simulink model "TractionControl"  (R2024b)
settings: Solver=FixedStepAuto  StartTime=0.0  StopTime=10.0  RelTol=1e-3  EnableMultiTasking=on
undefined symbols (not defined in the file): Ki1, rStraightSlipRatio, tSlipRatioDerivativeFilterCutoff, tTorqueControlTask
libraries: simulink x9
settings Model: DataDictionary=Master_Dictionary.sldd  EnableAccessToBaseWorkspace=off  Creator=torni  LastModifiedBy=Will
settings OptimizationCC: DefaultParameterBehavior=Inlined  EnhancedBackFolding=on  PassReuseOutputArgsAs=Individual arguments  ZeroExternalMemoryAtStartup=off  ZeroInternalMemoryAtStartup=off  MaxStackSize=8192  OptimizeBlockOrder=speed  DifferentSizesBufferReuse=on  OptimizationCustomize=off  EfficientTunableParamExpr=on
settings DebuggingCC: ParameterTunabilityLossMsg=error
settings HardwareCC: ProdBitPerPointer=32  ProdBitPerSizeT=32  ProdBitPerPtrDiffT=32  ProdLargestAtomicInteger=Long  ProdLargestAtomicFloat=Double  ProdWordSize=32  ProdLongLongMode=on  ProdHWDeviceType=ARM Compatible->ARM Cortex-M
settings SFSimCC: MATLABDynamicMemAlloc=off
settings RTWCC: Description=Embedded Coder  SystemTargetFile=ert.tlc  HardwareBoard=STM32H7xx Based (Single-core)  TemplateMakefile=ert_default_tmf  Toolchain=GNU Tools for ARM Embedded Processors
settings CodeAppCC: ForceParamTrailComments=on  IgnoreCustomStorageClasses=off  OperatorAnnotations=on  SimulinkDataObjDesc=on  SFDataObjDesc=on  InsertBlockDesc=on
settings ERTTargetCC: TargetLangStandard=C99 (ISO)  CodeReplacementLibrary=ARM Cortex-M  ExtModeTransport=3  ExtModeStaticAlloc=on  ExtModeStaticAllocSize=2048  ExtModeMexFile=ext_xcp  ExtModeIntrfLevel=Level2 - Open

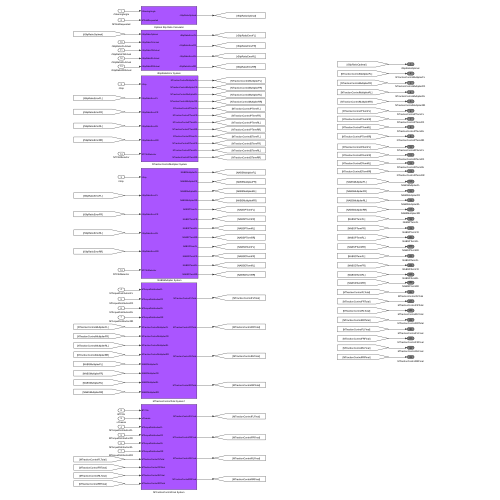
[thumbnail: Simulink's stored preview of the top-level diagram]
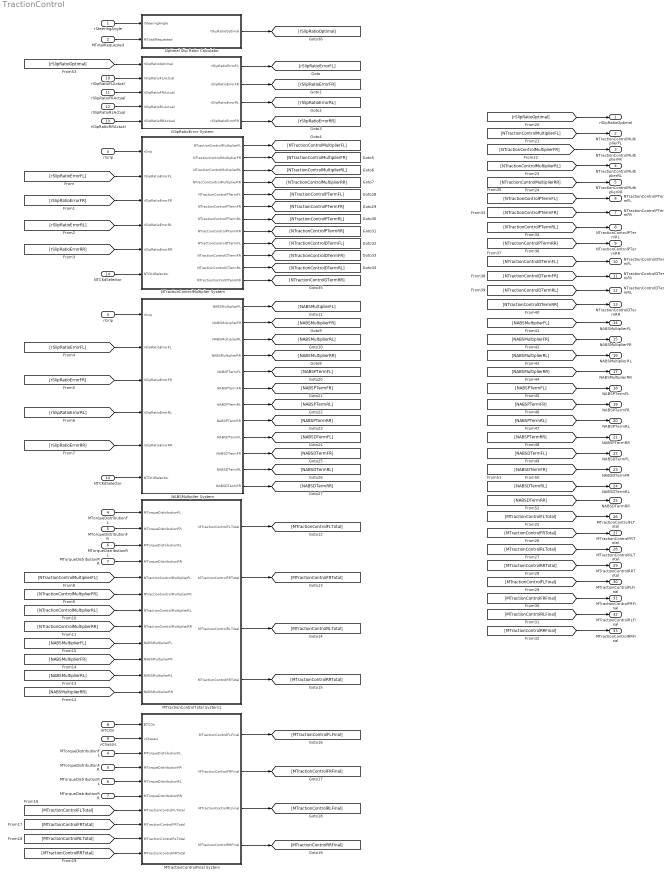
== system TractionControl ==
  rSteeringAngle : Inport
  MTotalRequested : Inport  Port=2
  rGrip : Inport  Port=3
  MTorqueDistributionFL : Inport  Port=4
  MTorqueDistributionFR : Inport  Port=5
  MTorqueDistributionRL : Inport  Port=6
  MTorqueDistributionRR : Inport  Port=7
  BTCOn : Inport  Port=8
  vChassis : Inport  Port=9
  rSlipRatioFLActual : Inport  Port=10
  rSlipRatioFRActual : Inport  Port=11
  rSlipRatioRLActual : Inport  Port=12
  rSlipRatioRRActual : Inport  Port=13
  NTCKdSelector : Inport  Port=14
  "MTorqueDistributionFL " : InportShadow  Port=4
  "MTorqueDistributionFR " : InportShadow  Port=5
  "MTorqueDistributionRL " : InportShadow  Port=6
  "MTorqueDistributionRR " : InportShadow  Port=7
  MTractionControlFinal System : Subsystem
  MTractionControlTotal System1 : Subsystem
  NABSMultiplier System : Subsystem
  "NTCKdSelector " : InportShadow  Port=14
  NTractionControlMultiplier System : Subsystem
  Optimal Slip Ratio Calculator : Subsystem
  "rGrip " : InportShadow  Port=3
  rSlipRatioError System : Subsystem
  "rSlipRatioOptimal " : Outport  VectorParamsAs1DForOutWhenUnconnected=off
  "NTractionControlMultiplierFL " : Outport  Port=2  VectorParamsAs1DForOutWhenUnconnected=off
  "NTractionControlMultiplierFR " : Outport  Port=3  VectorParamsAs1DForOutWhenUnconnected=off
  "NTractionControlMultiplierRL " : Outport  Port=4  VectorParamsAs1DForOutWhenUnconnected=off
  "NTractionControlMultiplierRR " : Outport  Port=5  VectorParamsAs1DForOutWhenUnconnected=off
  NTractionControlPTermFL : Outport  Port=6  VectorParamsAs1DForOutWhenUnconnected=off
  NTractionControlPTermFR : Outport  Port=7  VectorParamsAs1DForOutWhenUnconnected=off
  NTractionControlPTermRL : Outport  Port=8  VectorParamsAs1DForOutWhenUnconnected=off
  NTractionControlPTermRR : Outport  Port=9  VectorParamsAs1DForOutWhenUnconnected=off
  NTractionControlDTermFL : Outport  Port=10  VectorParamsAs1DForOutWhenUnconnected=off
  NTractionControlDTermFR : Outport  Port=11  VectorParamsAs1DForOutWhenUnconnected=off
  NTractionControlDTermRL : Outport  Port=12  VectorParamsAs1DForOutWhenUnconnected=off
  NTractionControlDTermRR : Outport  Port=13  VectorParamsAs1DForOutWhenUnconnected=off
  NABSMultiplierFL : Outport  Port=14  VectorParamsAs1DForOutWhenUnconnected=off
  NABSMultiplierFR : Outport  Port=15  VectorParamsAs1DForOutWhenUnconnected=off
  NABSMultiplierRL : Outport  Port=16  VectorParamsAs1DForOutWhenUnconnected=off
  NABSMultiplierRR : Outport  Port=17  VectorParamsAs1DForOutWhenUnconnected=off
  NABSPTermFL : Outport  Port=18  VectorParamsAs1DForOutWhenUnconnected=off
  NABSPTermFR : Outport  Port=19  VectorParamsAs1DForOutWhenUnconnected=off
  NABSPTermRL : Outport  Port=20  VectorParamsAs1DForOutWhenUnconnected=off
  NABSPTermRR : Outport  Port=21  VectorParamsAs1DForOutWhenUnconnected=off
  NABSDTermFL : Outport  Port=22  VectorParamsAs1DForOutWhenUnconnected=off
  NABSDTermFR : Outport  Port=23  VectorParamsAs1DForOutWhenUnconnected=off
  NABSDTermRL : Outport  Port=24  VectorParamsAs1DForOutWhenUnconnected=off
  NABSDTermRR : Outport  Port=25  VectorParamsAs1DForOutWhenUnconnected=off
  MTractionControlFLTotal : Outport  Port=26  VectorParamsAs1DForOutWhenUnconnected=off
  MTractionControlFRTotal : Outport  Port=27  VectorParamsAs1DForOutWhenUnconnected=off
  MTractionControlRLTotal : Outport  Port=28  VectorParamsAs1DForOutWhenUnconnected=off
  MTractionControlRRTotal : Outport  Port=29  VectorParamsAs1DForOutWhenUnconnected=off
  MTractionControlFLFinal : Outport  Port=30  VectorParamsAs1DForOutWhenUnconnected=off
  MTractionControlFRFinal : Outport  Port=31  VectorParamsAs1DForOutWhenUnconnected=off
  MTractionControlRLFinal : Outport  Port=32  VectorParamsAs1DForOutWhenUnconnected=off
  MTractionControlRRFinal : Outport  Port=33  VectorParamsAs1DForOutWhenUnconnected=off
  wires:
  rSteeringAngle/1 -> Optimal Slip Ratio Calculator/1(rSteeringAngle)
  MTotalRequested/1 -> Optimal Slip Ratio Calculator/2(MTotalRequested)
  rGrip/1 -> NTractionControlMultiplier System/1(rGrip)
  [rSlipRatioErrorFL] -> NTractionControlMultiplier System/2(rSlipRatioErrorFL)
  [rSlipRatioErrorFR] -> NTractionControlMultiplier System/3(rSlipRatioErrorFR)
  [rSlipRatioErrorRL] -> NTractionControlMultiplier System/4(rSlipRatioErrorRL)
  [rSlipRatioErrorRR] -> NTractionControlMultiplier System/5(rSlipRatioErrorRR)
  "rGrip "/1 -> NABSMultiplier System/1(rGrip)
  MTorqueDistributionFL/1 -> MTractionControlTotal System1/1(MTorqueDistributionFL)
  MTorqueDistributionFR/1 -> MTractionControlTotal System1/2(MTorqueDistributionFR)
  MTorqueDistributionRL/1 -> MTractionControlTotal System1/3(MTorqueDistributionRL)
  MTorqueDistributionRR/1 -> MTractionControlTotal System1/4(MTorqueDistributionRR)
  BTCOn/1 -> MTractionControlFinal System/1(BTCOn)
  vChassis/1 -> MTractionControlFinal System/2(vChassis)
  "MTorqueDistributionFL "/1 -> MTractionControlFinal System/3(MTorqueDistributionFL)
  "MTorqueDistributionFR "/1 -> MTractionControlFinal System/4(MTorqueDistributionFR)
  "MTorqueDistributionRL "/1 -> MTractionControlFinal System/5(MTorqueDistributionRL)
  "MTorqueDistributionRR "/1 -> MTractionControlFinal System/6(MTorqueDistributionRR)
  [rSlipRatioErrorFL] -> NABSMultiplier System/2(rSlipRatioErrorFL)
  [rSlipRatioErrorFR] -> NABSMultiplier System/3(rSlipRatioErrorFR)
  [rSlipRatioErrorRL] -> NABSMultiplier System/4(rSlipRatioErrorRL)
  [rSlipRatioErrorRR] -> NABSMultiplier System/5(rSlipRatioErrorRR)
  [NTractionControlMultiplierFL] -> MTractionControlTotal System1/5(NTractionControlMultiplierFL)
  [NTractionControlMultiplierFR] -> MTractionControlTotal System1/6(NTractionControlMultiplierFR)
  [NTractionControlMultiplierRL] -> MTractionControlTotal System1/7(NTractionControlMultiplierRL)
  [NTractionControlMultiplierRR] -> MTractionControlTotal System1/8(NTractionControlMultiplierRR)
  [NABSMultiplierRR] -> MTractionControlTotal System1/12(NABSMultiplierRR)
  [NABSMultiplierRL] -> MTractionControlTotal System1/11(NABSMultiplierRL)
  [NABSMultiplierFL] -> MTractionControlTotal System1/9(NABSMultiplierFL)
  [NABSMultiplierFR] -> MTractionControlTotal System1/10(NABSMultiplierFR)
  MTractionControlTotal System1/1(MTractionControlFLTotal) -> [MTractionControlFLTotal]
  [MTractionControlFLTotal] -> MTractionControlFinal System/7(MTractionControlFLTotal)
  [MTractionControlFRTotal] -> MTractionControlFinal System/8(MTractionControlFRTotal)
  MTractionControlTotal System1/2(MTractionControlFRTotal) -> [MTractionControlFRTotal]
  MTractionControlTotal System1/3(MTractionControlRLTotal) -> [MTractionControlRLTotal]
  [MTractionControlRLTotal] -> MTractionControlFinal System/9(MTractionControlRLTotal)
  MTractionControlTotal System1/4(MTractionControlRRTotal) -> [MTractionControlRRTotal]
  [MTractionControlRRTotal] -> MTractionControlFinal System/10(MTractionControlRRTotal)
  NTractionControlMultiplier System/1(NTractionControlMultiplierFL) -> [NTractionControlMultiplierFL]
  NTractionControlMultiplier System/2(NTractionControlMultiplierFR) -> [NTractionControlMultiplierFR]
  NTractionControlMultiplier System/3(NTractionControlMultiplierRL) -> [NTractionControlMultiplierRL]
  NTractionControlMultiplier System/4(NTractionControlMultiplierRR) -> [NTractionControlMultiplierRR]
  MTractionControlFinal System/1(MTractionControlFLFinal) -> [MTractionControlFLFinal]
  MTractionControlFinal System/2(MTractionControlFRFinal) -> [MTractionControlFRFinal]
  MTractionControlFinal System/3(MTractionControlRLFinal) -> [MTractionControlRLFinal]
  MTractionControlFinal System/4(MTractionControlRRFinal) -> [MTractionControlRRFinal]
  NABSMultiplier System/1(NABSMultiplierFL) -> [NABSMultiplierFL]
  NABSMultiplier System/2(NABSMultiplierFR) -> [NABSMultiplierFR]
  NABSMultiplier System/3(NABSMultiplierRL) -> [NABSMultiplierRL]
  NABSMultiplier System/4(NABSMultiplierRR) -> [NABSMultiplierRR]
  NABSMultiplier System/5(NABSPTermFL) -> [NABSPTermFL]
  NABSMultiplier System/6(NABSPTermFR) -> [NABSPTermFR]
  NABSMultiplier System/7(NABSPTermRL) -> [NABSPTermRL]
  NABSMultiplier System/8(NABSPTermRR) -> [NABSPTermRR]
  NABSMultiplier System/9(NABSDTermFL) -> [NABSDTermFL]
  NABSMultiplier System/10(NABSDTermFR) -> [NABSDTermFR]
  NABSMultiplier System/11(NABSDTermRL) -> [NABSDTermRL]
  NABSMultiplier System/12(NABSDTermRR) -> [NABSDTermRR]
  NTractionControlMultiplier System/5(NTractionControlPTermFL) -> [NTractionControlPTermFL]
  NTractionControlMultiplier System/6(NTractionControlPTermFR) -> [NTractionControlPTermFR]
  NTractionControlMultiplier System/7(NTractionControlPTermRL) -> [NTractionControlPTermRL]
  NTractionControlMultiplier System/8(NTractionControlPTermRR) -> [NTractionControlPTermRR]
  NTractionControlMultiplier System/9(NTractionControlDTermFL) -> [NTractionControlDTermFL]
  NTractionControlMultiplier System/10(NTractionControlDTermFR) -> [NTractionControlDTermFR]
  NTractionControlMultiplier System/11(NTractionControlDTermRL) -> [NTractionControlDTermRL]
  NTractionControlMultiplier System/12(NTractionControlDTermRR) -> [NTractionControlDTermRR]
  rSlipRatioError System/1(rSlipRatioErrorFL) -> [rSlipRatioErrorFL]
  rSlipRatioError System/2(rSlipRatioErrorFR) -> [rSlipRatioErrorFR]
  rSlipRatioError System/3(rSlipRatioErrorRL) -> [rSlipRatioErrorRL]
  rSlipRatioError System/4(rSlipRatioErrorRR) -> [rSlipRatioErrorRR]
  Optimal Slip Ratio Calculator/1(rSlipRatioOptimal) -> [rSlipRatioOptimal]
  [rSlipRatioOptimal] -> rSlipRatioError System/1(rSlipRatioOptimal)
  rSlipRatioFLActual/1 -> rSlipRatioError System/2("rSlipRatioFLActual ")
  rSlipRatioFRActual/1 -> rSlipRatioError System/3("rSlipRatioFRActual ")
  rSlipRatioRLActual/1 -> rSlipRatioError System/4("rSlipRatioRLActual ")
  rSlipRatioRRActual/1 -> rSlipRatioError System/5("rSlipRatioRRActual ")
  [rSlipRatioOptimal] -> "rSlipRatioOptimal "/1
  [NTractionControlMultiplierFL] -> "NTractionControlMultiplierFL "/1
  [NTractionControlMultiplierRL] -> "NTractionControlMultiplierRL "/1
  [NTractionControlMultiplierFR] -> "NTractionControlMultiplierFR "/1
  [NTractionControlMultiplierRR] -> "NTractionControlMultiplierRR "/1
  [NTractionControlPTermFL] -> NTractionControlPTermFL/1
  [NTractionControlPTermFR] -> NTractionControlPTermFR/1
  [NTractionControlPTermRR] -> NTractionControlPTermRR/1
  [NTractionControlPTermRL] -> NTractionControlPTermRL/1
  [NTractionControlDTermFL] -> NTractionControlDTermFL/1
  [NTractionControlDTermFR] -> NTractionControlDTermFR/1
  [NTractionControlDTermRL] -> NTractionControlDTermRL/1
  [NTractionControlDTermRR] -> NTractionControlDTermRR/1
  [NABSMultiplierFL] -> NABSMultiplierFL/1
  [NABSMultiplierFR] -> NABSMultiplierFR/1
  [NABSMultiplierRL] -> NABSMultiplierRL/1
  [NABSMultiplierRR] -> NABSMultiplierRR/1
  [NABSPTermFL] -> NABSPTermFL/1
  [NABSPTermFR] -> NABSPTermFR/1
  [NABSPTermRL] -> NABSPTermRL/1
  [NABSPTermRR] -> NABSPTermRR/1
  [NABSDTermFL] -> NABSDTermFL/1
  [NABSDTermFR] -> NABSDTermFR/1
  [NABSDTermRL] -> NABSDTermRL/1
  [NABSDTermRR] -> NABSDTermRR/1
  [MTractionControlFLTotal] -> MTractionControlFLTotal/1
  [MTractionControlFLFinal] -> MTractionControlFLFinal/1
  [MTractionControlRRTotal] -> MTractionControlRRTotal/1
  [MTractionControlRLTotal] -> MTractionControlRLTotal/1
  [MTractionControlFRTotal] -> MTractionControlFRTotal/1
  [MTractionControlFRFinal] -> MTractionControlFRFinal/1
  [MTractionControlRLFinal] -> MTractionControlRLFinal/1
  [MTractionControlRRFinal] -> MTractionControlRRFinal/1
  NTCKdSelector/1 -> NTractionControlMultiplier System/6(NTCKdSelector)
  "NTCKdSelector "/1 -> NABSMultiplier System/6(NTCKdSelector)

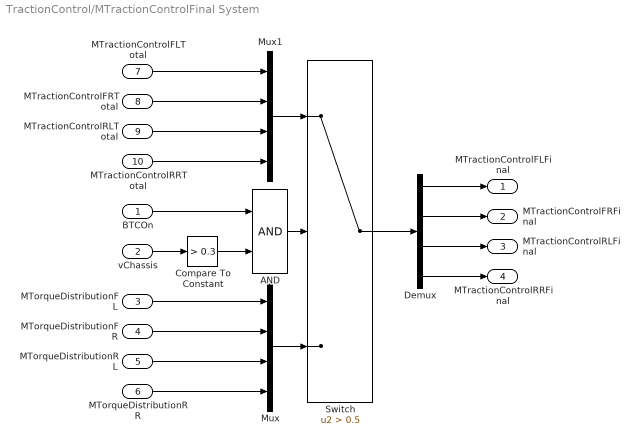
== system TractionControl/MTractionControlFinal System ==
  BTCOn : Inport  OutDataTypeStr=boolean
  vChassis : Inport  Port=2  OutDataTypeStr=double
  MTorqueDistributionFL : Inport  Port=3  OutDataTypeStr=double
  MTorqueDistributionFR : Inport  Port=4  OutDataTypeStr=double
  MTorqueDistributionRL : Inport  Port=5  OutDataTypeStr=double
  MTorqueDistributionRR : Inport  Port=6  OutDataTypeStr=double
  MTractionControlFLTotal : Inport  Port=7  OutDataTypeStr=double
  MTractionControlFRTotal : Inport  Port=8  OutDataTypeStr=double
  MTractionControlRLTotal : Inport  Port=9  OutDataTypeStr=double
  MTractionControlRRTotal : Inport  Port=10  OutDataTypeStr=double
  AND : Logic  AllPortsSameDT=off  OutDataTypeStr=boolean
  Compare To Constant : simulink/Logic and Bit Operations/Compare To Constant  relop=>  const=0.3  OutDataTypeStr=boolean
  Demux : Demux
  Mux : Mux
  Mux1 : Mux
  Switch : Switch  Criteria=u2 > Threshold  Threshold=0.5  SaturateOnIntegerOverflow=off  InputSameDT=off
  MTractionControlFLFinal : Outport  OutDataTypeStr=double  VectorParamsAs1DForOutWhenUnconnected=off
  MTractionControlFRFinal : Outport  Port=2  OutDataTypeStr=double  VectorParamsAs1DForOutWhenUnconnected=off
  MTractionControlRLFinal : Outport  Port=3  OutDataTypeStr=double  VectorParamsAs1DForOutWhenUnconnected=off
  MTractionControlRRFinal : Outport  Port=4  OutDataTypeStr=double  VectorParamsAs1DForOutWhenUnconnected=off
  wires:
  Mux1/1 -> Switch/1
  Demux/4 -> MTractionControlRRFinal/1
  MTractionControlFRTotal/1 -> Mux1/2
  MTractionControlRLTotal/1 -> Mux1/3
  Compare To Constant/1 -> AND/2
  Demux/3 -> MTractionControlRLFinal/1
  MTorqueDistributionFL/1 -> Mux/1
  MTractionControlFLTotal/1 -> Mux1/1
  MTractionControlRRTotal/1 -> Mux1/4
  AND/1 -> Switch/2
  Demux/1 -> MTractionControlFLFinal/1
  Switch/1 -> Demux/1
  MTorqueDistributionFR/1 -> Mux/2
  MTorqueDistributionRR/1 -> Mux/4
  vChassis/1 -> Compare To Constant/1
  Mux/1 -> Switch/3
  MTorqueDistributionRL/1 -> Mux/3
  Demux/2 -> MTractionControlFRFinal/1
  BTCOn/1 -> AND/1

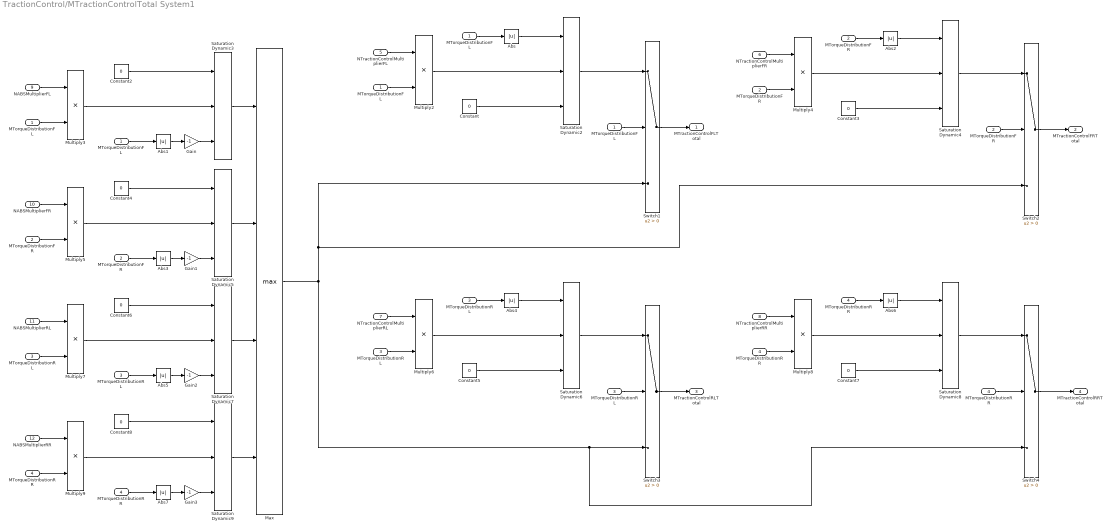
== system TractionControl/MTractionControlTotal System1 ==
  MTorqueDistributionFL : Inport  OutDataTypeStr=double
  MTorqueDistributionFR : Inport  Port=2  OutDataTypeStr=double
  MTorqueDistributionRL : Inport  Port=3  OutDataTypeStr=double
  MTorqueDistributionRR : Inport  Port=4  OutDataTypeStr=double
  NTractionControlMultiplierFL : Inport  Port=5  OutDataTypeStr=double
  NTractionControlMultiplierFR : Inport  Port=6  OutDataTypeStr=double
  NTractionControlMultiplierRL : Inport  Port=7  OutDataTypeStr=double
  NTractionControlMultiplierRR : Inport  Port=8  OutDataTypeStr=double
  NABSMultiplierFL : Inport  Port=9  OutDataTypeStr=double
  NABSMultiplierFR : Inport  Port=10  OutDataTypeStr=double
  NABSMultiplierRL : Inport  Port=11  OutDataTypeStr=double
  NABSMultiplierRR : Inport  Port=12  OutDataTypeStr=double
  Abs{,1..7} (8 alike) : Abs  SaturateOnIntegerOverflow=off
  Constant{,2..8} (8 alike) : Constant  Value=0
  Gain{,1..3} (4 alike) : Gain  Gain=-1
  "MTorqueDistributionFL " : InportShadow  OutDataTypeStr=double
  "MTorqueDistributionFL " : InportShadow  OutDataTypeStr=double
  "MTorqueDistributionFL   " : InportShadow  OutDataTypeStr=double
  "MTorqueDistributionFL    " : InportShadow  OutDataTypeStr=double
  "MTorqueDistributionFR " : InportShadow  Port=2  OutDataTypeStr=double
  "MTorqueDistributionFR " : InportShadow  Port=2  OutDataTypeStr=double
  "MTorqueDistributionFR   " : InportShadow  Port=2  OutDataTypeStr=double
  "MTorqueDistributionFR    " : InportShadow  Port=2  OutDataTypeStr=double
  "MTorqueDistributionRL " : InportShadow  Port=3  OutDataTypeStr=double
  "MTorqueDistributionRL " : InportShadow  Port=3  OutDataTypeStr=double
  "MTorqueDistributionRL   " : InportShadow  Port=3  OutDataTypeStr=double
  "MTorqueDistributionRL    " : InportShadow  Port=3  OutDataTypeStr=double
  "MTorqueDistributionRR " : InportShadow  Port=4  OutDataTypeStr=double
  "MTorqueDistributionRR " : InportShadow  Port=4  OutDataTypeStr=double
  "MTorqueDistributionRR   " : InportShadow  Port=4  OutDataTypeStr=double
  "MTorqueDistributionRR    " : InportShadow  Port=4  OutDataTypeStr=double
  Max : MinMax  Function=max  Inputs=4
  Multiply{2..9} (8 alike) : Product
  Saturation Dynamic{2..9} (8 alike) : simulink/Discontinuities/Saturation Dynamic  OutMin=[]  OutMax=[]  OutDataTypeStr=Inherit: Same as second input  OutDataType=fixdt(1, 16)  OutScaling=2^-10  DoSatur=off
  Switch{1..4} (4 alike) : Switch  Criteria=u2 > Threshold  SaturateOnIntegerOverflow=off  InputSameDT=off
  MTractionControlFLTotal : Outport  OutDataTypeStr=double  VectorParamsAs1DForOutWhenUnconnected=off
  MTractionControlFRTotal : Outport  Port=2  OutDataTypeStr=double  VectorParamsAs1DForOutWhenUnconnected=off
  MTractionControlRLTotal : Outport  Port=3  OutDataTypeStr=double  VectorParamsAs1DForOutWhenUnconnected=off
  MTractionControlRRTotal : Outport  Port=4  OutDataTypeStr=double  VectorParamsAs1DForOutWhenUnconnected=off
  wires:
  Switch1/1 -> MTractionControlFLTotal/1
  Saturation Dynamic2/1 -> Switch1/1
  "MTorqueDistributionFL "/1 -> Abs/1
  Constant/1 -> Saturation Dynamic2/3
  Multiply2/1 -> Saturation Dynamic2/2
  NTractionControlMultiplierFL/1 -> Multiply2/1
  MTorqueDistributionFL/1 -> Multiply2/2
  "MTorqueDistributionFL    "/1 -> Switch1/2
  Saturation Dynamic3/1 -> Max/1
  Constant2/1 -> Saturation Dynamic3/1
  "MTorqueDistributionFL "/1 -> Abs1/1
  Abs/1 -> Saturation Dynamic2/1
  Abs1/1 -> Gain/1
  Gain/1 -> Saturation Dynamic3/3
  Multiply3/1 -> Saturation Dynamic3/2
  NABSMultiplierFL/1 -> Multiply3/1
  "MTorqueDistributionFL   "/1 -> Multiply3/2
  "MTorqueDistributionFR   "/1 -> Multiply5/2
  NABSMultiplierFR/1 -> Multiply5/1
  Multiply5/1 -> Saturation Dynamic5/2
  Gain1/1 -> Saturation Dynamic5/3
  Abs3/1 -> Gain1/1
  Abs2/1 -> Saturation Dynamic4/1
  "MTorqueDistributionFR "/1 -> Abs3/1
  Constant4/1 -> Saturation Dynamic5/1
  "MTorqueDistributionFR    "/1 -> Switch2/2
  NTractionControlMultiplierFR/1 -> Multiply4/1
  Multiply4/1 -> Saturation Dynamic4/2
  Constant3/1 -> Saturation Dynamic4/3
  "MTorqueDistributionFR "/1 -> Abs2/1
  Saturation Dynamic4/1 -> Switch2/1
  Switch2/1 -> MTractionControlFRTotal/1
  MTorqueDistributionFR/1 -> Multiply4/2
  MTorqueDistributionRL/1 -> Multiply6/2
  Switch3/1 -> MTractionControlRLTotal/1
  Saturation Dynamic6/1 -> Switch3/1
  "MTorqueDistributionRL "/1 -> Abs4/1
  Constant5/1 -> Saturation Dynamic6/3
  Multiply6/1 -> Saturation Dynamic6/2
  NTractionControlMultiplierRL/1 -> Multiply6/1
  "MTorqueDistributionRL    "/1 -> Switch3/2
  Constant6/1 -> Saturation Dynamic7/1
  "MTorqueDistributionRL "/1 -> Abs5/1
  Abs4/1 -> Saturation Dynamic6/1
  Abs5/1 -> Gain2/1
  Gain2/1 -> Saturation Dynamic7/3
  Multiply7/1 -> Saturation Dynamic7/2
  NABSMultiplierRL/1 -> Multiply7/1
  "MTorqueDistributionRL   "/1 -> Multiply7/2
  "MTorqueDistributionRR   "/1 -> Multiply9/2
  NABSMultiplierRR/1 -> Multiply9/1
  Multiply9/1 -> Saturation Dynamic9/2
  Gain3/1 -> Saturation Dynamic9/3
  Abs7/1 -> Gain3/1
  Abs6/1 -> Saturation Dynamic8/1
  "MTorqueDistributionRR "/1 -> Abs7/1
  Constant8/1 -> Saturation Dynamic9/1
  "MTorqueDistributionRR    "/1 -> Switch4/2
  NTractionControlMultiplierRR/1 -> Multiply8/1
  Multiply8/1 -> Saturation Dynamic8/2
  Constant7/1 -> Saturation Dynamic8/3
  "MTorqueDistributionRR "/1 -> Abs6/1
  Saturation Dynamic8/1 -> Switch4/1
  Switch4/1 -> MTractionControlRRTotal/1
  MTorqueDistributionRR/1 -> Multiply8/2
  Saturation Dynamic5/1 -> Max/2
  Saturation Dynamic7/1 -> Max/3
  Saturation Dynamic9/1 -> Max/4
  Max/1 -> Switch4/3, Switch3/3, Switch2/3, Switch1/3

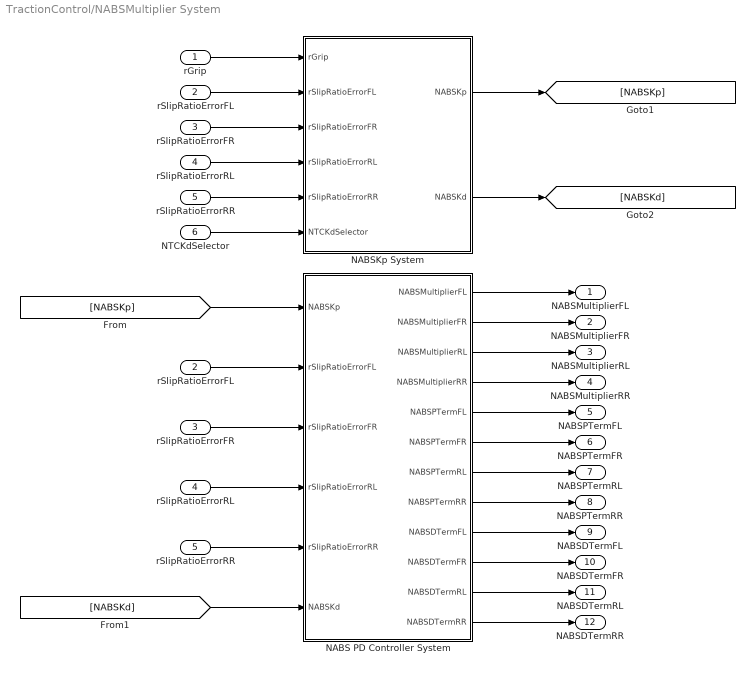
== system TractionControl/NABSMultiplier System ==
  rGrip : Inport
  rSlipRatioErrorFL : Inport  Port=2
  rSlipRatioErrorFR : Inport  Port=3
  rSlipRatioErrorRL : Inport  Port=4
  rSlipRatioErrorRR : Inport  Port=5
  NTCKdSelector : Inport  Port=6
  NABS PD Controller System : Subsystem
  NABSKp System : Subsystem
  "rSlipRatioErrorFL " : InportShadow  Port=2
  "rSlipRatioErrorFR " : InportShadow  Port=3
  "rSlipRatioErrorRL " : InportShadow  Port=4
  "rSlipRatioErrorRR " : InportShadow  Port=5
  NABSMultiplierFL : Outport  VectorParamsAs1DForOutWhenUnconnected=off
  NABSMultiplierFR : Outport  Port=2  VectorParamsAs1DForOutWhenUnconnected=off
  NABSMultiplierRL : Outport  Port=3  VectorParamsAs1DForOutWhenUnconnected=off
  NABSMultiplierRR : Outport  Port=4  VectorParamsAs1DForOutWhenUnconnected=off
  NABSPTermFL : Outport  Port=5  VectorParamsAs1DForOutWhenUnconnected=off
  NABSPTermFR : Outport  Port=6  VectorParamsAs1DForOutWhenUnconnected=off
  NABSPTermRL : Outport  Port=7  VectorParamsAs1DForOutWhenUnconnected=off
  NABSPTermRR : Outport  Port=8  VectorParamsAs1DForOutWhenUnconnected=off
  NABSDTermFL : Outport  Port=9  VectorParamsAs1DForOutWhenUnconnected=off
  NABSDTermFR : Outport  Port=10  VectorParamsAs1DForOutWhenUnconnected=off
  NABSDTermRL : Outport  Port=11  VectorParamsAs1DForOutWhenUnconnected=off
  NABSDTermRR : Outport  Port=12  VectorParamsAs1DForOutWhenUnconnected=off
  wires:
  [NABSKp] -> NABS PD Controller System/1(NABSKp)
  NABSKp System/1(NABSKp) -> [NABSKp]
  "rSlipRatioErrorFL "/1 -> NABS PD Controller System/2("rSlipRatioErrorFL ")
  "rSlipRatioErrorFR "/1 -> NABS PD Controller System/3(rSlipRatioErrorFR)
  "rSlipRatioErrorRL "/1 -> NABS PD Controller System/4(rSlipRatioErrorRL)
  "rSlipRatioErrorRR "/1 -> NABS PD Controller System/5(rSlipRatioErrorRR)
  NABS PD Controller System/1(NABSMultiplierFL) -> NABSMultiplierFL/1
  NABS PD Controller System/2(NABSMultiplierFR) -> NABSMultiplierFR/1
  NABS PD Controller System/3(NABSMultiplierRL) -> NABSMultiplierRL/1
  NABS PD Controller System/4(NABSMultiplierRR) -> NABSMultiplierRR/1
  NABS PD Controller System/5(NABSPTermFL) -> NABSPTermFL/1
  NABS PD Controller System/6(NABSPTermFR) -> NABSPTermFR/1
  NABS PD Controller System/7(NABSPTermRL) -> NABSPTermRL/1
  NABS PD Controller System/8(NABSPTermRR) -> NABSPTermRR/1
  NABS PD Controller System/9("NABSDTermFL ") -> NABSDTermFL/1
  NABS PD Controller System/10(NABSDTermFR) -> NABSDTermFR/1
  NABS PD Controller System/11(NABSDTermRL) -> NABSDTermRL/1
  NABS PD Controller System/12(NABSDTermRR) -> NABSDTermRR/1
  rSlipRatioErrorFL/1 -> NABSKp System/2(rSlipRatioErrorFL)
  rGrip/1 -> NABSKp System/1("rGrip ")
  rSlipRatioErrorRL/1 -> NABSKp System/4(rSlipRatioErrorRL)
  rSlipRatioErrorFR/1 -> NABSKp System/3(rSlipRatioErrorFR)
  rSlipRatioErrorRR/1 -> NABSKp System/5(rSlipRatioErrorRR)
  NABSKp System/2(NABSKd) -> [NABSKd]
  NTCKdSelector/1 -> NABSKp System/6(NTCKdSelector)
  [NABSKd] -> NABS PD Controller System/6(NABSKd)

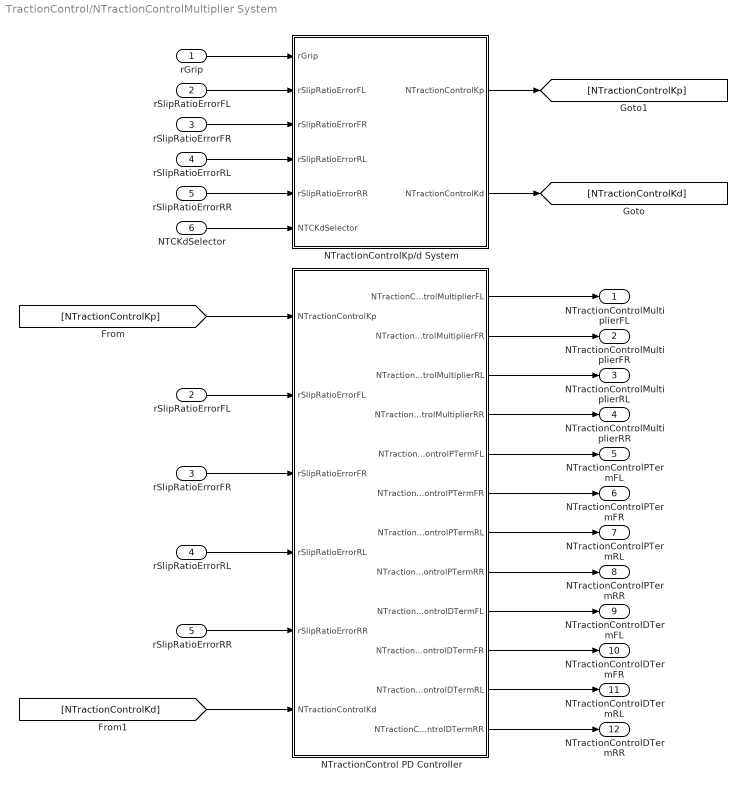
== system TractionControl/NTractionControlMultiplier System ==
  rGrip : Inport
  rSlipRatioErrorFL : Inport  Port=2
  rSlipRatioErrorFR : Inport  Port=3
  rSlipRatioErrorRL : Inport  Port=4
  rSlipRatioErrorRR : Inport  Port=5
  NTCKdSelector : Inport  Port=6
  NTractionControl PD Controller : Subsystem
  NTractionControlKp/d System : Subsystem
  "rSlipRatioErrorFL " : InportShadow  Port=2
  "rSlipRatioErrorFR " : InportShadow  Port=3
  "rSlipRatioErrorRL " : InportShadow  Port=4
  "rSlipRatioErrorRR " : InportShadow  Port=5
  NTractionControlMultiplierFL : Outport  VectorParamsAs1DForOutWhenUnconnected=off
  NTractionControlMultiplierFR : Outport  Port=2  VectorParamsAs1DForOutWhenUnconnected=off
  NTractionControlMultiplierRL : Outport  Port=3  VectorParamsAs1DForOutWhenUnconnected=off
  NTractionControlMultiplierRR : Outport  Port=4  VectorParamsAs1DForOutWhenUnconnected=off
  NTractionControlPTermFL : Outport  Port=5  VectorParamsAs1DForOutWhenUnconnected=off
  NTractionControlPTermFR : Outport  Port=6  VectorParamsAs1DForOutWhenUnconnected=off
  NTractionControlPTermRL : Outport  Port=7  VectorParamsAs1DForOutWhenUnconnected=off
  NTractionControlPTermRR : Outport  Port=8  VectorParamsAs1DForOutWhenUnconnected=off
  NTractionControlDTermFL : Outport  Port=9  VectorParamsAs1DForOutWhenUnconnected=off
  NTractionControlDTermFR : Outport  Port=10  VectorParamsAs1DForOutWhenUnconnected=off
  NTractionControlDTermRL : Outport  Port=11  VectorParamsAs1DForOutWhenUnconnected=off
  NTractionControlDTermRR : Outport  Port=12  VectorParamsAs1DForOutWhenUnconnected=off
  wires:
  NTractionControlKp/d System/1(NTractionControlKp) -> [NTractionControlKp]
  [NTractionControlKp] -> NTractionControl PD Controller/1(NTractionControlKp)
  rGrip/1 -> NTractionControlKp/d System/1("rGrip ")
  rSlipRatioErrorFL/1 -> NTractionControlKp/d System/2(rSlipRatioErrorFL)
  rSlipRatioErrorFR/1 -> NTractionControlKp/d System/3(rSlipRatioErrorFR)
  rSlipRatioErrorRR/1 -> NTractionControlKp/d System/5(rSlipRatioErrorRR)
  rSlipRatioErrorRL/1 -> NTractionControlKp/d System/4(rSlipRatioErrorRL)
  "rSlipRatioErrorFL "/1 -> NTractionControl PD Controller/2("rSlipRatioErrorFL ")
  "rSlipRatioErrorFR "/1 -> NTractionControl PD Controller/3(rSlipRatioErrorFR)
  "rSlipRatioErrorRL "/1 -> NTractionControl PD Controller/4(rSlipRatioErrorRL)
  "rSlipRatioErrorRR "/1 -> NTractionControl PD Controller/5(rSlipRatioErrorRR)
  NTractionControl PD Controller/1(NTractionControlMultiplierFL) -> NTractionControlMultiplierFL/1
  NTractionControl PD Controller/2(NTractionControlMultiplierFR) -> NTractionControlMultiplierFR/1
  NTractionControl PD Controller/3(NTractionControlMultiplierRL) -> NTractionControlMultiplierRL/1
  NTractionControl PD Controller/4(NTractionControlMultiplierRR) -> NTractionControlMultiplierRR/1
  NTractionControl PD Controller/5(NTractionControlPTermFL) -> NTractionControlPTermFL/1
  NTractionControl PD Controller/6(NTractionControlPTermFR) -> NTractionControlPTermFR/1
  NTractionControl PD Controller/7(NTractionControlPTermRL) -> NTractionControlPTermRL/1
  NTractionControl PD Controller/8(NTractionControlPTermRR) -> NTractionControlPTermRR/1
  NTractionControl PD Controller/9("NTractionControlDTermFL ") -> NTractionControlDTermFL/1
  NTractionControl PD Controller/10(NTractionControlDTermFR) -> NTractionControlDTermFR/1
  NTractionControl PD Controller/11(NTractionControlDTermRL) -> NTractionControlDTermRL/1
  NTractionControl PD Controller/12(NTractionControlDTermRR) -> NTractionControlDTermRR/1
  [NTractionControlKd] -> NTractionControl PD Controller/6(NTractionControlKd)
  NTCKdSelector/1 -> NTractionControlKp/d System/6(NTCKdSelector)
  NTractionControlKp/d System/2(NTractionControlKd) -> [NTractionControlKd]

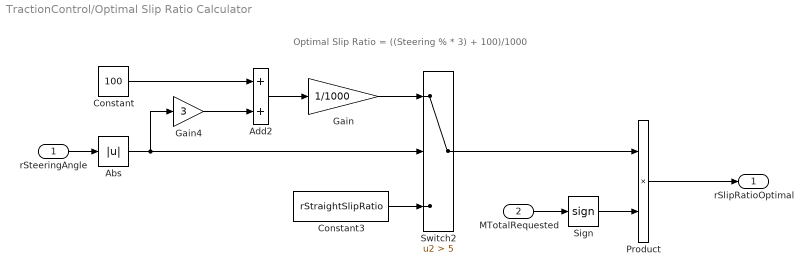
== system TractionControl/Optimal Slip Ratio Calculator ==
  note: Optimal Slip Ratio = ((Steering % * 3) + 100)/1000
  rSteeringAngle : Inport  OutDataTypeStr=double
  MTotalRequested : Inport  Port=2  OutDataTypeStr=double
  Abs : Abs  SaturateOnIntegerOverflow=off
  Add2 : Sum
  Constant : Constant  Value=100
  Constant3 : Constant  Value=rStraightSlipRatio
  Gain : Gain  Gain=1/1000
  Gain4 : Gain  Gain=3
  Product : Product
  Sign : Signum
  Switch2 : Switch  Criteria=u2 > Threshold  Threshold=5  SaturateOnIntegerOverflow=off  InputSameDT=off
  rSlipRatioOptimal : Outport  OutDataTypeStr=double  VectorParamsAs1DForOutWhenUnconnected=off
  wires:
  Sign/1 -> Product/2
  Constant/1 -> Add2/1
  MTotalRequested/1 -> Sign/1
  Gain4/1 -> Add2/2
  Product/1 -> rSlipRatioOptimal/1
  Switch2/1 -> Product/1
  Abs/1 -> Gain4/1, Switch2/2
  Constant3/1 -> Switch2/3
  rSteeringAngle/1 -> Abs/1
  Add2/1 -> Gain/1
  Gain/1 -> Switch2/1

== system TractionControl/rSlipRatioError System ==
  rSlipRatioOptimal : Inport  OutDataTypeStr=double
  "rSlipRatioFLActual " : Inport  Port=2  OutDataTypeStr=double
  "rSlipRatioFRActual " : Inport  Port=3  OutDataTypeStr=double
  "rSlipRatioRLActual " : Inport  Port=4  OutDataTypeStr=double
  "rSlipRatioRRActual " : Inport  Port=5  OutDataTypeStr=double
  Demux : Demux
  Mux : Mux
  Subtract : Sum  Inputs=+-
  rSlipRatioErrorFL : Outport  VectorParamsAs1DForOutWhenUnconnected=off
  rSlipRatioErrorFR : Outport  Port=2  VectorParamsAs1DForOutWhenUnconnected=off
  rSlipRatioErrorRL : Outport  Port=3  VectorParamsAs1DForOutWhenUnconnected=off
  rSlipRatioErrorRR : Outport  Port=4  VectorParamsAs1DForOutWhenUnconnected=off
  wires:
  Demux/1 -> rSlipRatioErrorFL/1
  Demux/2 -> rSlipRatioErrorFR/1
  Demux/3 -> rSlipRatioErrorRL/1
  Demux/4 -> rSlipRatioErrorRR/1
  Subtract/1 -> Demux/1
  "rSlipRatioFLActual "/1 -> Mux/1
  "rSlipRatioFRActual "/1 -> Mux/2
  Mux/1 -> Subtract/1
  "rSlipRatioRLActual "/1 -> Mux/3
  "rSlipRatioRRActual "/1 -> Mux/4
  rSlipRatioOptimal/1 -> Subtract/2

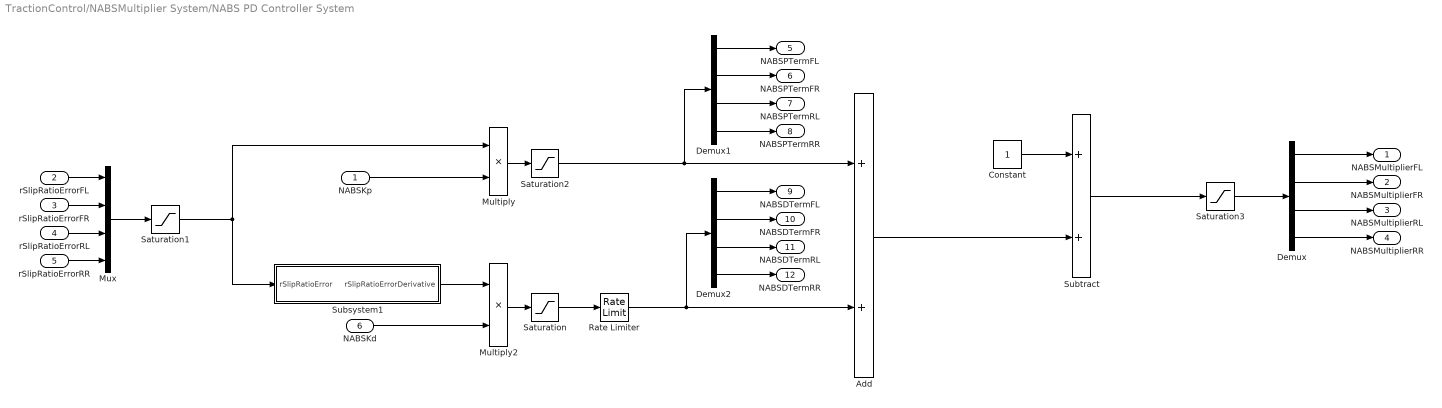
== system TractionControl/NABSMultiplier System/NABS PD Controller System ==
  NABSKp : Inport
  "rSlipRatioErrorFL " : Inport  Port=2
  rSlipRatioErrorFR : Inport  Port=3
  rSlipRatioErrorRL : Inport  Port=4
  rSlipRatioErrorRR : Inport  Port=5
  NABSKd : Inport  Port=6
  Add : Sum
  Constant : Constant
  Demux : Demux
  Demux1 : Demux
  Demux2 : Demux
  Multiply : Product
  Multiply2 : Product
  Mux : Mux
  Rate Limiter : RateLimiter  RisingSlewLimit=30  FallingSlewLimit=-6  SampleTimeMode=inherited
  Saturation : Saturate  LowerLimit=0
  Saturation1 : Saturate  UpperLimit=1  LowerLimit=-1
  Saturation2 : Saturate  UpperLimit=0  LowerLimit=-2
  Saturation3 : Saturate  UpperLimit=1  LowerLimit=0
  Subsystem1 : Subsystem
  Subtract : Sum
  NABSMultiplierFL : Outport  OutDataTypeStr=double  VectorParamsAs1DForOutWhenUnconnected=off
  NABSMultiplierFR : Outport  Port=2  OutDataTypeStr=double  VectorParamsAs1DForOutWhenUnconnected=off
  NABSMultiplierRL : Outport  Port=3  OutDataTypeStr=double  VectorParamsAs1DForOutWhenUnconnected=off
  NABSMultiplierRR : Outport  Port=4  OutDataTypeStr=double  VectorParamsAs1DForOutWhenUnconnected=off
  NABSPTermFL : Outport  Port=5  VectorParamsAs1DForOutWhenUnconnected=off
  NABSPTermFR : Outport  Port=6  VectorParamsAs1DForOutWhenUnconnected=off
  NABSPTermRL : Outport  Port=7  VectorParamsAs1DForOutWhenUnconnected=off
  NABSPTermRR : Outport  Port=8  VectorParamsAs1DForOutWhenUnconnected=off
  "NABSDTermFL " : Outport  Port=9  VectorParamsAs1DForOutWhenUnconnected=off
  NABSDTermFR : Outport  Port=10  VectorParamsAs1DForOutWhenUnconnected=off
  NABSDTermRL : Outport  Port=11  VectorParamsAs1DForOutWhenUnconnected=off
  NABSDTermRR : Outport  Port=12  VectorParamsAs1DForOutWhenUnconnected=off
  wires:
  Demux1/2 -> NABSPTermFR/1
  Saturation1/1 -> Subsystem1/1(rSlipRatioError), Multiply/1
  Add/1 -> Subtract/2
  Subtract/1 -> Saturation3/1
  Multiply2/1 -> Saturation/1
  Demux2/3 -> NABSDTermRL/1
  Demux2/1 -> "NABSDTermFL "/1
  "rSlipRatioErrorFL "/1 -> Mux/1
  Constant/1 -> Subtract/1
  Demux1/1 -> NABSPTermFL/1
  Saturation2/1 -> Demux1/1, Add/1
  Saturation3/1 -> Demux/1
  Demux2/4 -> NABSDTermRR/1
  Demux2/2 -> NABSDTermFR/1
  Demux1/3 -> NABSPTermRL/1
  rSlipRatioErrorRR/1 -> Mux/4
  Demux1/4 -> NABSPTermRR/1
  Subsystem1/1(rSlipRatioErrorDerivative) -> Multiply2/1
  Demux/2 -> NABSMultiplierFR/1
  Demux/1 -> NABSMultiplierFL/1
  Demux/3 -> NABSMultiplierRL/1
  NABSKp/1 -> Multiply/2
  Mux/1 -> Saturation1/1
  rSlipRatioErrorRL/1 -> Mux/3
  Multiply/1 -> Saturation2/1
  rSlipRatioErrorFR/1 -> Mux/2
  NABSKd/1 -> Multiply2/2
  Saturation/1 -> Rate Limiter/1
  Rate Limiter/1 -> Demux2/1, Add/2
  Demux/4 -> NABSMultiplierRR/1

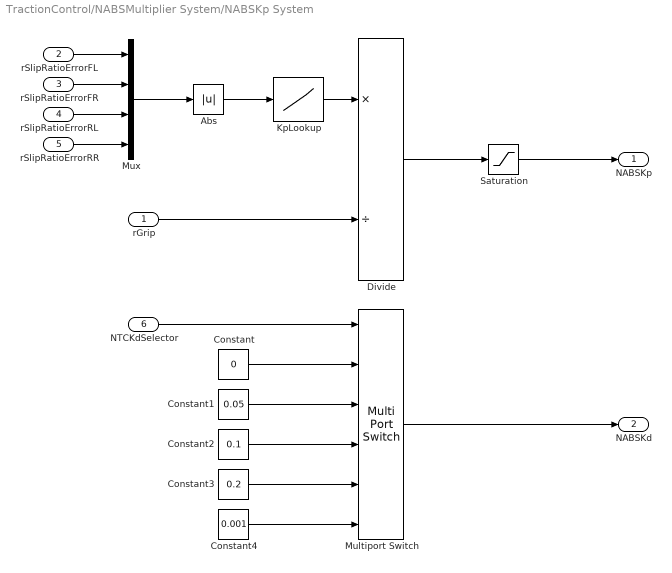
== system TractionControl/NABSMultiplier System/NABSKp System ==
  "rGrip " : Inport
  rSlipRatioErrorFL : Inport  Port=2
  rSlipRatioErrorFR : Inport  Port=3
  rSlipRatioErrorRL : Inport  Port=4
  rSlipRatioErrorRR : Inport  Port=5
  NTCKdSelector : Inport  Port=6
  Abs : Abs  SaturateOnIntegerOverflow=off
  Constant : Constant  Value=0
  Constant1 : Constant  Value=0.05
  Constant2 : Constant  Value=0.1
  Constant3 : Constant  Value=0.2
  Constant4 : Constant  Value=0.001
  Divide : Product  Inputs=*/
  KpLookup : Lookup_n-D  NumberOfTableDimensions=1  BreakpointsForDimension1=[0,0.1,0.11,0.12,0.13,0.14,0.15,0.16,0.17,0.18,0.19,0.2,0.21,0.22,0.23,0.24,0.25,0.26,0.27,0.28,0.29,0.3,0.31,0.32,0.33,0.34,0.35,0.36,0.37,0.38,0.39,0.4,0.41,0.42,0.43,0.44,0.45,0.46,0.47,0.48,0.49,0.5]  BreakpointsForDimension2=Ki1  Table=[0.1,0.1,0.1175,0.135,0.1525,0.17,0.1875,0.205,0.2225,0.24,0.2575,0.275,0.2925,0.31,0.3275,0.345,0.3625,0.38,0.3975,0.415,0.4325,0.45,0.4675,0.485,0.5025,0.52,0.5375,0.555,0.5725,0.59,0.6075,0.625,0.6425,0.66,0.6775,0.695,0.7125,0.73,0.7475,0.765,0.7825,0.8]  InternalRulePriority=Speed  RndMeth=Simplest
  Multiport Switch : MultiPortSwitch  Inputs=5  SaturateOnIntegerOverflow=off  InputSameDT=off
  Mux : Mux
  Saturation : Saturate  UpperLimit=2  LowerLimit=0
  NABSKp : Outport  OutDataTypeStr=double  VectorParamsAs1DForOutWhenUnconnected=off
  NABSKd : Outport  Port=2  OutDataTypeStr=double  VectorParamsAs1DForOutWhenUnconnected=off
  wires:
  rSlipRatioErrorFL/1 -> Mux/1
  rSlipRatioErrorFR/1 -> Mux/2
  Abs/1 -> KpLookup/1
  Mux/1 -> Abs/1
  KpLookup/1 -> Divide/1
  Divide/1 -> Saturation/1
  Saturation/1 -> NABSKp/1
  "rGrip "/1 -> Divide/2
  rSlipRatioErrorRR/1 -> Mux/4
  rSlipRatioErrorRL/1 -> Mux/3
  Multiport Switch/1 -> NABSKd/1
  NTCKdSelector/1 -> Multiport Switch/1
  Constant/1 -> Multiport Switch/2
  Constant1/1 -> Multiport Switch/3
  Constant2/1 -> Multiport Switch/4
  Constant3/1 -> Multiport Switch/5
  Constant4/1 -> Multiport Switch/6

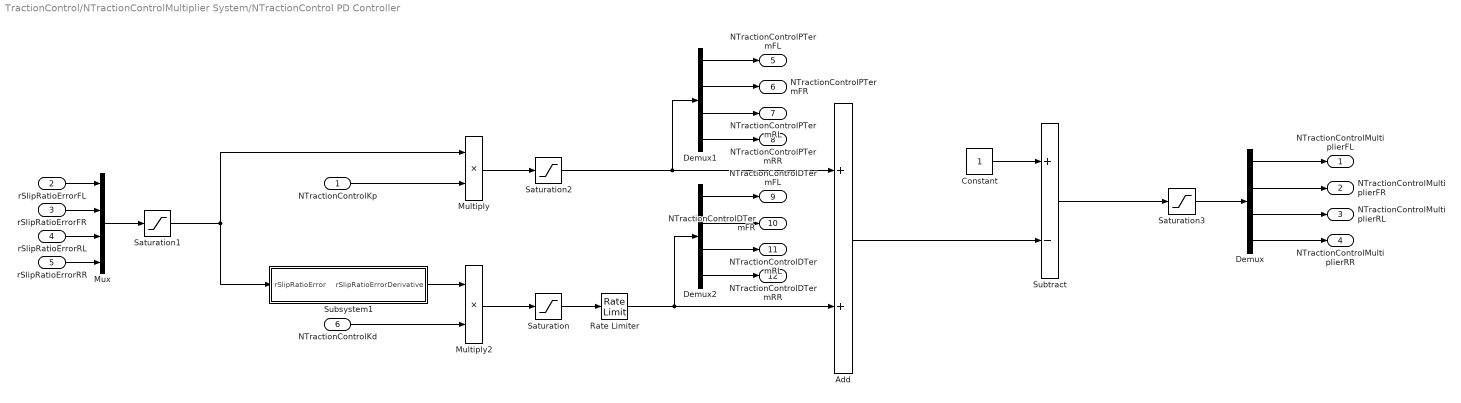
== system TractionControl/NTractionControlMultiplier System/NTractionControl PD Controller ==
  NTractionControlKp : Inport
  "rSlipRatioErrorFL " : Inport  Port=2
  rSlipRatioErrorFR : Inport  Port=3
  rSlipRatioErrorRL : Inport  Port=4
  rSlipRatioErrorRR : Inport  Port=5
  NTractionControlKd : Inport  Port=6
  Add : Sum
  Constant : Constant
  Demux : Demux
  Demux1 : Demux
  Demux2 : Demux
  Multiply : Product
  Multiply2 : Product
  Mux : Mux
  Rate Limiter : RateLimiter  RisingSlewLimit=6  FallingSlewLimit=-30  SampleTimeMode=inherited
  Saturation : Saturate  UpperLimit=0
  Saturation1 : Saturate  UpperLimit=1  LowerLimit=-1
  Saturation2 : Saturate  UpperLimit=2  LowerLimit=0
  Saturation3 : Saturate  UpperLimit=1  LowerLimit=0
  Subsystem1 : Subsystem
  Subtract : Sum  Inputs=+-
  NTractionControlMultiplierFL : Outport  OutDataTypeStr=double  VectorParamsAs1DForOutWhenUnconnected=off
  NTractionControlMultiplierFR : Outport  Port=2  OutDataTypeStr=double  VectorParamsAs1DForOutWhenUnconnected=off
  NTractionControlMultiplierRL : Outport  Port=3  OutDataTypeStr=double  VectorParamsAs1DForOutWhenUnconnected=off
  NTractionControlMultiplierRR : Outport  Port=4  OutDataTypeStr=double  VectorParamsAs1DForOutWhenUnconnected=off
  NTractionControlPTermFL : Outport  Port=5  VectorParamsAs1DForOutWhenUnconnected=off
  NTractionControlPTermFR : Outport  Port=6  VectorParamsAs1DForOutWhenUnconnected=off
  NTractionControlPTermRL : Outport  Port=7  VectorParamsAs1DForOutWhenUnconnected=off
  NTractionControlPTermRR : Outport  Port=8  VectorParamsAs1DForOutWhenUnconnected=off
  "NTractionControlDTermFL " : Outport  Port=9  VectorParamsAs1DForOutWhenUnconnected=off
  NTractionControlDTermFR : Outport  Port=10  VectorParamsAs1DForOutWhenUnconnected=off
  NTractionControlDTermRL : Outport  Port=11  VectorParamsAs1DForOutWhenUnconnected=off
  NTractionControlDTermRR : Outport  Port=12  VectorParamsAs1DForOutWhenUnconnected=off
  wires:
  NTractionControlKd/1 -> Multiply2/2
  Multiply/1 -> Saturation2/1
  Demux/2 -> NTractionControlMultiplierFR/1
  Demux1/3 -> NTractionControlPTermRL/1
  Saturation2/1 -> Demux1/1, Add/1
  Subsystem1/1(rSlipRatioErrorDerivative) -> Multiply2/1
  Demux2/4 -> NTractionControlDTermRR/1
  Demux1/1 -> NTractionControlPTermFL/1
  Demux2/3 -> NTractionControlDTermRL/1
  Demux2/1 -> "NTractionControlDTermFL "/1
  Saturation1/1 -> Multiply/1, Subsystem1/1(rSlipRatioError)
  Demux/4 -> NTractionControlMultiplierRR/1
  rSlipRatioErrorFR/1 -> Mux/2
  Demux/3 -> NTractionControlMultiplierRL/1
  rSlipRatioErrorRL/1 -> Mux/3
  Demux1/4 -> NTractionControlPTermRR/1
  rSlipRatioErrorRR/1 -> Mux/4
  Demux2/2 -> NTractionControlDTermFR/1
  Multiply2/1 -> Saturation/1
  "rSlipRatioErrorFL "/1 -> Mux/1
  Constant/1 -> Subtract/1
  NTractionControlKp/1 -> Multiply/2
  Demux1/2 -> NTractionControlPTermFR/1
  Saturation/1 -> Rate Limiter/1
  Saturation3/1 -> Demux/1
  Add/1 -> Subtract/2
  Subtract/1 -> Saturation3/1
  Demux/1 -> NTractionControlMultiplierFL/1
  Rate Limiter/1 -> Demux2/1, Add/2
  Mux/1 -> Saturation1/1

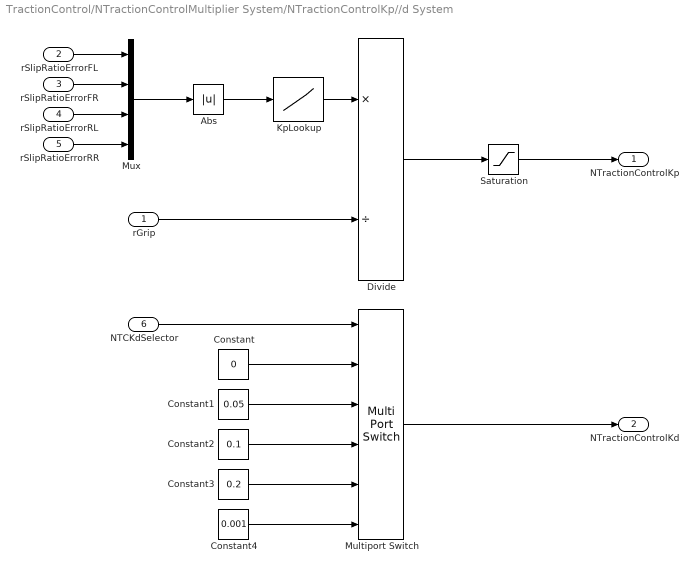
== system TractionControl/NTractionControlMultiplier System/NTractionControlKp//d System ==
  "rGrip " : Inport
  rSlipRatioErrorFL : Inport  Port=2
  rSlipRatioErrorFR : Inport  Port=3
  rSlipRatioErrorRL : Inport  Port=4
  rSlipRatioErrorRR : Inport  Port=5
  NTCKdSelector : Inport  Port=6
  Abs : Abs  SaturateOnIntegerOverflow=off
  Constant : Constant  Value=0
  Constant1 : Constant  Value=0.05
  Constant2 : Constant  Value=0.1
  Constant3 : Constant  Value=0.2
  Constant4 : Constant  Value=0.001
  Divide : Product  Inputs=*/
  KpLookup : Lookup_n-D  NumberOfTableDimensions=1  BreakpointsForDimension1=[0,0.1,0.11,0.12,0.13,0.14,0.15,0.16,0.17,0.18,0.19,0.2,0.21,0.22,0.23,0.24,0.25,0.26,0.27,0.28,0.29,0.3,0.31,0.32,0.33,0.34,0.35,0.36,0.37,0.38,0.39,0.4,0.41,0.42,0.43,0.44,0.45,0.46,0.47,0.48,0.49,0.5]  BreakpointsForDimension2=Ki1  Table=[0.1,0.1,0.1175,0.135,0.1525,0.17,0.1875,0.205,0.2225,0.24,0.2575,0.275,0.2925,0.31,0.3275,0.345,0.3625,0.38,0.3975,0.415,0.4325,0.45,0.4675,0.485,0.5025,0.52,0.5375,0.555,0.5725,0.59,0.6075,0.625,0.6425,0.66,0.6775,0.695,0.7125,0.73,0.7475,0.765,0.7825,0.8]  InternalRulePriority=Speed  RndMeth=Simplest
  Multiport Switch : MultiPortSwitch  Inputs=5  SaturateOnIntegerOverflow=off  InputSameDT=off
  Mux : Mux
  Saturation : Saturate  UpperLimit=2  LowerLimit=0
  NTractionControlKp : Outport  OutDataTypeStr=double  VectorParamsAs1DForOutWhenUnconnected=off
  NTractionControlKd : Outport  Port=2  OutDataTypeStr=double  VectorParamsAs1DForOutWhenUnconnected=off
  wires:
  rSlipRatioErrorFL/1 -> Mux/1
  rSlipRatioErrorFR/1 -> Mux/2
  Abs/1 -> KpLookup/1
  Mux/1 -> Abs/1
  KpLookup/1 -> Divide/1
  Divide/1 -> Saturation/1
  Saturation/1 -> NTractionControlKp/1
  "rGrip "/1 -> Divide/2
  rSlipRatioErrorRR/1 -> Mux/4
  rSlipRatioErrorRL/1 -> Mux/3
  Multiport Switch/1 -> NTractionControlKd/1
  NTCKdSelector/1 -> Multiport Switch/1
  Constant/1 -> Multiport Switch/2
  Constant1/1 -> Multiport Switch/3
  Constant2/1 -> Multiport Switch/4
  Constant3/1 -> Multiport Switch/5
  Constant4/1 -> Multiport Switch/6

== system TractionControl/NABSMultiplier System/NABS PD Controller System/Subsystem1 ==
  rSlipRatioError : Inport  OutDataTypeStr=double
  Add : Sum  Inputs=+-
  Gain : Gain  Gain=1/0.001
  Low Pass Filter : Subsystem
  Memory : Memory  InheritSampleTime=on
  y(k-1) : Memory  InheritSampleTime=on
  rSlipRatioErrorDerivative : Outport  VectorParamsAs1DForOutWhenUnconnected=off
  wires:
  Add/1 -> Gain/1
  Memory/1 -> Add/2
  rSlipRatioError/1 -> Memory/1, Add/1
  Gain/1 -> Low Pass Filter/1(u(k)), y(k-1)/1  "u(k)"
  y(k-1)/1 -> Low Pass Filter/2(y(k-1))
  Low Pass Filter/1(rSlipRatioErrorDerivative) -> rSlipRatioErrorDerivative/1

== system TractionControl/NTractionControlMultiplier System/NTractionControl PD Controller/Subsystem1 ==
  rSlipRatioError : Inport  OutDataTypeStr=double
  Add : Sum  Inputs=+-
  Gain : Gain  Gain=1/0.001
  Low Pass Filter : Subsystem
  Memory : Memory  InheritSampleTime=on
  y(k-1) : Memory  InheritSampleTime=on
  rSlipRatioErrorDerivative : Outport  VectorParamsAs1DForOutWhenUnconnected=off
  wires:
  Add/1 -> Gain/1
  Memory/1 -> Add/2
  rSlipRatioError/1 -> Memory/1, Add/1
  Gain/1 -> Low Pass Filter/1(u(k)), y(k-1)/1  "u(k)"
  y(k-1)/1 -> Low Pass Filter/2(y(k-1))
  Low Pass Filter/1(rSlipRatioErrorDerivative) -> rSlipRatioErrorDerivative/1

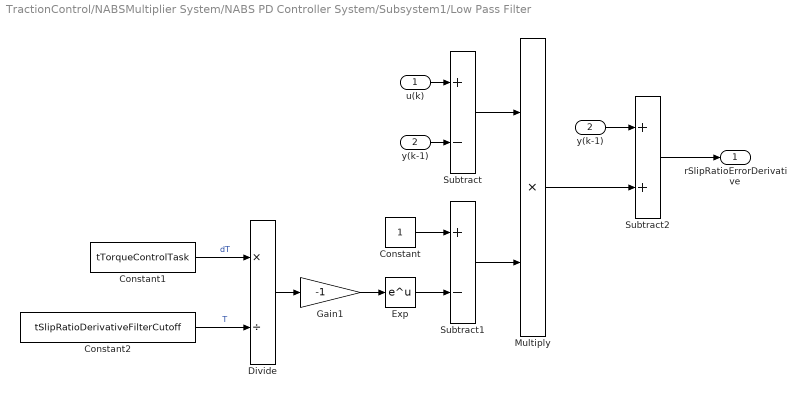
== system TractionControl/NABSMultiplier System/NABS PD Controller System/Subsystem1/Low Pass Filter ==
  u(k) : Inport
  y(k-1) : Inport  Port=2
  Constant : Constant
  Constant1 : Constant  Value=tTorqueControlTask
  Constant2 : Constant  Value=tSlipRatioDerivativeFilterCutoff
  Divide : Product  Inputs=*/  RndMeth=Zero  SaturateOnIntegerOverflow=on
  Exp : Math  SignedPower=on
  Gain1 : Gain  Gain=-1
  Multiply : Product
  Subtract : Sum  Inputs=+-
  Subtract1 : Sum  Inputs=+-
  Subtract2 : Sum
  "y(k-1) " : InportShadow  Port=2
  rSlipRatioErrorDerivative : Outport  VectorParamsAs1DForOutWhenUnconnected=off
  wires:
  Divide/1 -> Gain1/1
  Subtract2/1 -> rSlipRatioErrorDerivative/1
  Constant2/1 -> Divide/2  "T"
  Subtract/1 -> Multiply/1
  Constant1/1 -> Divide/1  "dT"
  Constant/1 -> Subtract1/1
  Subtract1/1 -> Multiply/2
  Multiply/1 -> Subtract2/2
  Exp/1 -> Subtract1/2
  Gain1/1 -> Exp/1
  u(k)/1 -> Subtract/1
  "y(k-1) "/1 -> Subtract2/1
  y(k-1)/1 -> Subtract/2

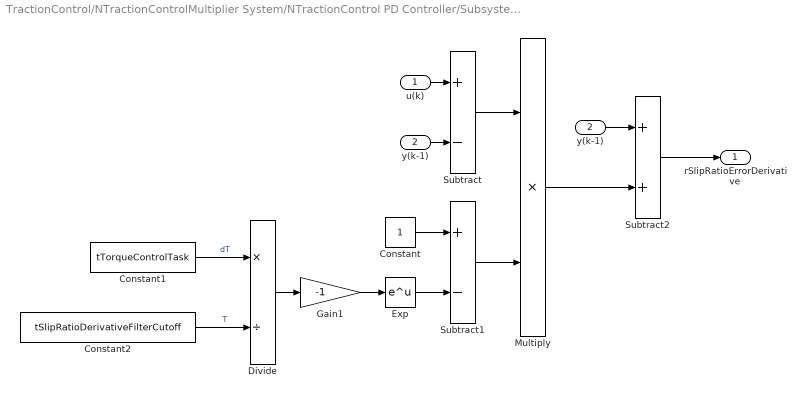
== system TractionControl/NTractionControlMultiplier System/NTractionControl PD Controller/Subsystem1/Low Pass Filter ==
  u(k) : Inport
  y(k-1) : Inport  Port=2
  Constant : Constant
  Constant1 : Constant  Value=tTorqueControlTask
  Constant2 : Constant  Value=tSlipRatioDerivativeFilterCutoff
  Divide : Product  Inputs=*/  RndMeth=Zero  SaturateOnIntegerOverflow=on
  Exp : Math  SignedPower=on
  Gain1 : Gain  Gain=-1
  Multiply : Product
  Subtract : Sum  Inputs=+-
  Subtract1 : Sum  Inputs=+-
  Subtract2 : Sum
  "y(k-1) " : InportShadow  Port=2
  rSlipRatioErrorDerivative : Outport  VectorParamsAs1DForOutWhenUnconnected=off
  wires:
  Divide/1 -> Gain1/1
  Subtract2/1 -> rSlipRatioErrorDerivative/1
  Constant2/1 -> Divide/2  "T"
  Subtract/1 -> Multiply/1
  Constant1/1 -> Divide/1  "dT"
  Constant/1 -> Subtract1/1
  Subtract1/1 -> Multiply/2
  Multiply/1 -> Subtract2/2
  Exp/1 -> Subtract1/2
  Gain1/1 -> Exp/1
  u(k)/1 -> Subtract/1
  "y(k-1) "/1 -> Subtract2/1
  y(k-1)/1 -> Subtract/2
